simulink model "dc_motor"  (R2020a)
settings: Solver=FixedStepAuto  StartTime=0.0  StopTime=300  FixedStep=ts  RelTol=1e-3
values from neighbouring files (symbols this model uses):
  J = 0.08    [Saving_the_data.m]    (also in parameters_of_dc_motor.m)
  K = 0.139    [Saving_the_data.m]    (also in parameters_of_dc_motor.m)
  L = 0.44    [Saving_the_data.m]    (also in parameters_of_dc_motor.m)
  Re = 2.4    [Saving_the_data.m]    (also in parameters_of_dc_motor.m)
  Rm = 0.01    [Saving_the_data.m]    (also in parameters_of_dc_motor.m)
  Tc = 0.1    [parameters_of_dc_motor.m]
  Ua = 120    [Saving_the_data.m]    (also in parameters_of_dc_motor.m = 40)
undefined symbols (not defined in the file or in its folder): sigbuilder_block
settings Model: Creator=Asus  LastModifiedBy=Asus

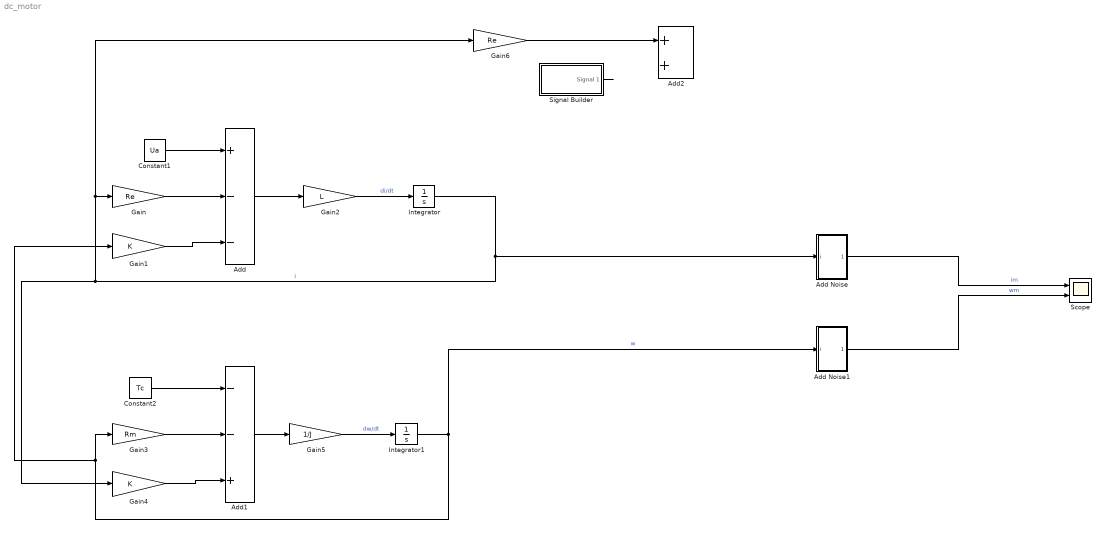
== system dc_motor ==
  Add : Sum  Inputs=+--
  Add Noise : Subsystem
  Add Noise1 : Subsystem
  Add1 : Sum  Inputs=--+
  Add2 : Sum
  Constant1 : Constant  Value=Ua
  Constant2 : Constant  Value=Tc
  Gain : Gain  Gain=Re
  Gain1 : Gain  Gain=K
  Gain2 : Gain  Gain=L
  Gain3 : Gain  Gain=Rm
  Gain4 : Gain  Gain=K
  Gain5 : Gain  Gain=1/J
  Gain6 : Gain  Gain=Re
  Integrator : Integrator
  Integrator1 : Integrator
  Scope : Scope  NumInputPorts=2
  Signal Builder : Subsystem  Tag=STV Subsys  LoadFcn=sigbuilder_block('load',[437.6 199.2 550.4 400 ]);  StartFcn=sigbuilder_block('start');  StopFcn=sigbuilder_block('stop');  ClipboardFcn=sigbuilder_block('clipboard');  mask(Sigbuilder block){tuvar=[0:10]}
      mask help: Simulink:masks:SigbuilderBlock_MD
      mask init:
      | if ~strcmp(get_param(bdroot(gcbh),'SimulationStatus'),'stopped') tuvar = sigbuilder_block('maskInit'); end
      settings: CopyFcn=sigbuilder_block('copy');  DeleteFcn=sigbuilder_block('delete');  ModelCloseFcn=sigbuilder_block('modelClose');  PreSaveFcn=sigbuilder_block('preSave');  PauseFcn=sigbuilder_block('pause');  ContinueFcn=sigbuilder_block('continue');  NameChangeFcn=sigbuilder_block('namechange');  OpenFcn=sigbuilder_block('open',[437.6 199.2 550.4 400 ]);  CloseFcn=sigbuilder_block('close');
      mask Display: plot(0, 0, 100, 100,[2, 2, 32, 32, 2], [68, 8, 8, 68, 68],[32, 2], [38, 38], [32, 19, 2],[53, 60, 44], [32, 17, 17, 2],[16, 16, 31, 31]);txt = getActiveGroup(gcbh);text(2, 100, txt,'verticalAlignment', 'top');
  wires:
  Constant1/1 -> Add/1
  Gain/1 -> Add/2
  Gain1/1 -> Add/3
  Add/1 -> Gain2/1
  Gain2/1 -> Integrator/1  "di/dt"
  Integrator/1 -> Gain4/1, Gain6/1, Gain/1, Add Noise/1(i)  "i"
  Constant2/1 -> Add1/1
  Gain3/1 -> Add1/2
  Gain4/1 -> Add1/3
  Add1/1 -> Gain5/1
  Gain5/1 -> Integrator1/1  "dw/dt"
  Integrator1/1 -> Add Noise1/1(i), Gain1/1, Gain3/1  "w"
  Add Noise/1(Out1) -> Scope/1  "im"
  Add Noise1/1(Out1) -> Scope/2  "wm"
  Gain6/1 -> Add2/1
  Signal Builder/1(Signal 1) -> ?

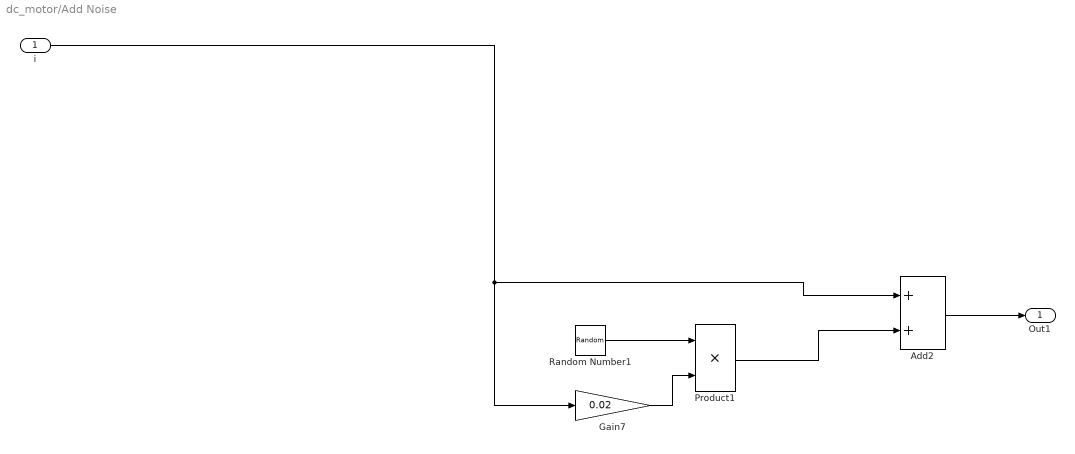
== system dc_motor/Add Noise ==
  i : Inport
  Add2 : Sum
  Gain7 : Gain  Gain=0.02
  Product1 : Product
  Random Number1 : RandomNumber  SampleTime=0.1
  Out1 : Outport
  wires:
  i/1 -> Gain7/1, Add2/1
  Add2/1 -> Out1/1
  Gain7/1 -> Product1/2
  Product1/1 -> Add2/2
  Random Number1/1 -> Product1/1

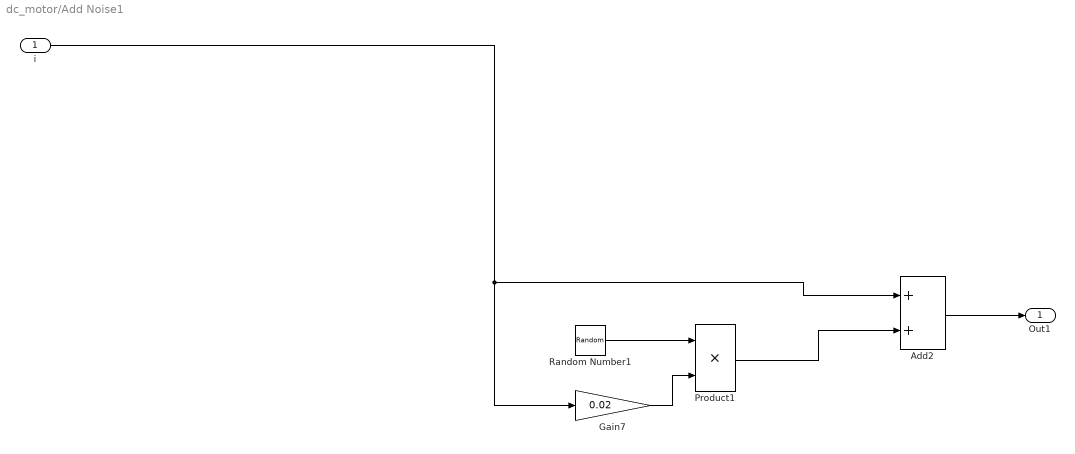
== system dc_motor/Add Noise1 ==
  i : Inport
  Add2 : Sum
  Gain7 : Gain  Gain=0.02
  Product1 : Product
  Random Number1 : RandomNumber  SampleTime=0.1
  Out1 : Outport
  wires:
  Random Number1/1 -> Product1/1
  Product1/1 -> Add2/2
  Gain7/1 -> Product1/2
  Add2/1 -> Out1/1
  i/1 -> Add2/1, Gain7/1

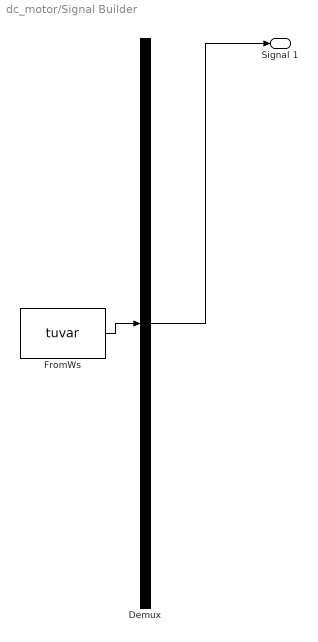
== system dc_motor/Signal Builder ==
  Demux : Demux  Tag=STV Demux  Outputs=1
      settings: DisplayOption=none
  FromWs : FromWorkspace  Tag=STV FromWs  VariableName=tuvar
      SigBuilderData=|
      | common.afterFinalStr = 'Extrapolate'
      | common.sampleTime = 0
      | dataSet.timeRange = [0 300]
      | dataSet.name = 'Group 1'
      | sbobj.Groups.Name = 'Group 1'
      | sbobj.Groups.Signals.Name = 'Signal 1'
      | sbobj.Groups.Signals.XData = [0 99.5 100 200 201 300]
      | sbobj.Groups.Signals.YData = [0 0 0.4 0.4 0 0]
      | sbobj.Groups.TimeRange = [0 300]
  Signal 1 : Outport  Tag=STV Outport
  wires:
  Demux/1 -> Signal 1/1
  FromWs/1 -> Demux/1
